simulink model "ExRobotAndEnvironmentControllerContPI"  (Simulink 8.9)
settings: Solver=ode45  StartTime=0.0  StopTime=1000  FixedStep=.01  RelTol=1e-3  EnableMultiTasking=on
undefined symbols (not defined in the file): Env, INITIAL_ROBOT_POS_THETA, INITIAL_ROBOT_POS_X, INITIAL_ROBOT_POS_Y, INTER_WHEEL_DISTANCE, ki_teta, kp_teta, MAX_SPEED, Robot, RobotInit, T, threshold_blanc, threshold_distance, threshold_noir, ts, ts_anim
libraries: simulink x3
settings Model: SuppressorTable=22 serialization::archive 11 0 6 0 0 0 11 0  Creator=alex  LastModifiedBy=esperonb  NumberOfSteps=100
settings OptimizationCC: ExpressionDepthLimit=2147483647
settings SFSimCC: SimParseCustomCode=off

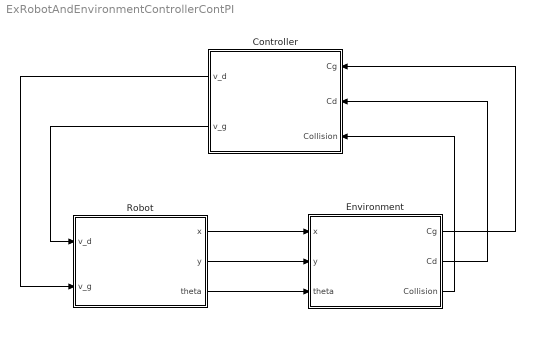
== system ExRobotAndEnvironmentControllerContPI ==
  Controller : Subsystem
  Environment : Subsystem
  Robot : Subsystem
  wires:
  Robot/1(x) -> Environment/1(x)
  Robot/2(y) -> Environment/2(y)
  Robot/3(theta) -> Environment/3(theta)
  Environment/1(Cg) -> Controller/1(Cg)
  Environment/2(Cd) -> Controller/2(Cd)
  Controller/1(v_d) -> Robot/2(v_g)
  Controller/2(v_g) -> Robot/1(v_d)
  Environment/3("Collision ") -> Controller/3("Collision ")

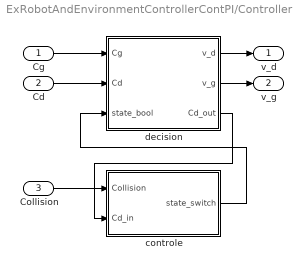
== system ExRobotAndEnvironmentControllerContPI/Controller ==
  Cg : Inport  OutDataTypeStr=double
  Cd : Inport  Port=2  OutDataTypeStr=double
  "Collision " : Inport  Port=3
  controle : Subsystem
  decision : Subsystem
  v_d : Outport
  v_g : Outport  Port=2
  wires:
  "Collision "/1 -> controle/1("Collision ")
  decision/3(Cd_out) -> controle/2(Cd_in)
  controle/1("state_switch ") -> decision/3("state_bool ")
  Cg/1 -> decision/1(Cg)
  Cd/1 -> decision/2(Cd)
  decision/1(v_d) -> v_d/1
  decision/2(v_g) -> v_g/1

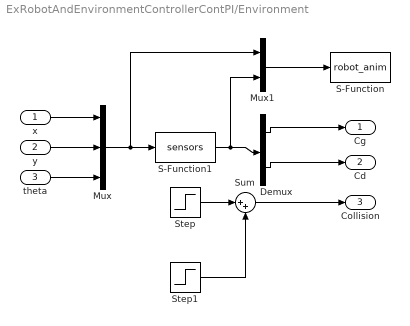
== system ExRobotAndEnvironmentControllerContPI/Environment ==
  x : Inport
  y : Inport  Port=2
  theta : Inport  Port=3
  Demux : Demux  Outputs=2
  Mux : Mux  Inputs=3
  Mux1 : Mux  Inputs=2
  S-Function : S-Function  FunctionName=robot_anim  Parameters=ts_anim,Env,Robot,RobotInit  SFunctionDeploymentMode=off  EnableBusSupport=off
  S-Function1 : S-Function  FunctionName=sensors  Parameters=ts,Env,Robot  SFunctionDeploymentMode=off  EnableBusSupport=off
  Step : Step  Time=2  SampleTime=0
  Step1 : Step  Time=2.1  After=-1  SampleTime=0
  Sum : Sum  Inputs=|++
  Cg : Outport  OutDataTypeStr=double
  Cd : Outport  Port=2
  "Collision " : Outport  Port=3
  wires:
  x/1 -> Mux/1
  y/1 -> Mux/2
  theta/1 -> Mux/3
  Mux/1 -> S-Function1/1, Mux1/1
  S-Function1/1 -> Mux1/2, Demux/1
  Mux1/1 -> S-Function/1
  Demux/1 -> Cg/1
  Demux/2 -> Cd/1
  Sum/1 -> "Collision "/1
  Step/1 -> Sum/1
  Step1/1 -> Sum/2

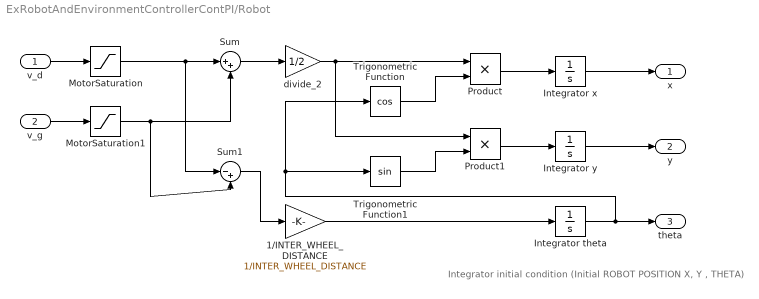
== system ExRobotAndEnvironmentControllerContPI/Robot ==
  note: Integrator initial condition (Initial ROBOT POSITION X, Y , THETA)
  v_d : Inport
  v_g : Inport  Port=2
  1/INTER_WHEEL_DISTANCE : Gain  Gain=1/INTER_WHEEL_DISTANCE
  Integrator theta : Integrator  InitialCondition=INITIAL_ROBOT_POS_THETA
  Integrator x : Integrator  InitialCondition=INITIAL_ROBOT_POS_X
  Integrator y : Integrator  InitialCondition=INITIAL_ROBOT_POS_Y
  MotorSaturation : Saturate  UpperLimit=MAX_SPEED  LowerLimit=-MAX_SPEED
  MotorSaturation1 : Saturate  UpperLimit=MAX_SPEED  LowerLimit=-MAX_SPEED
  Product : Product  RndMeth=Zero
  Product1 : Product  RndMeth=Zero
  Sum : Sum  Inputs=|++
  Sum1 : Sum  Inputs=|-+
  Trigonometric Function : Trigonometry  Operator=cos
  Trigonometric Function1 : Trigonometry
  divide_2 : Gain  Gain=1/2
  x : Outport
  y : Outport  Port=2
  theta : Outport  Port=3
  wires:
  v_d/1 -> MotorSaturation/1
  Integrator x/1 -> x/1
  Integrator y/1 -> y/1
  Integrator theta/1 -> Trigonometric Function/1, Trigonometric Function1/1, theta/1
  Sum/1 -> divide_2/1
  divide_2/1 -> Product1/1, Product/1
  Trigonometric Function/1 -> Product/2
  Trigonometric Function1/1 -> Product1/2
  Product/1 -> Integrator x/1
  Product1/1 -> Integrator y/1
  Sum1/1 -> 1/INTER_WHEEL_DISTANCE/1
  1/INTER_WHEEL_DISTANCE/1 -> Integrator theta/1
  v_g/1 -> MotorSaturation1/1
  MotorSaturation1/1 -> Sum/2, Sum1/2
  MotorSaturation/1 -> Sum/1, Sum1/1

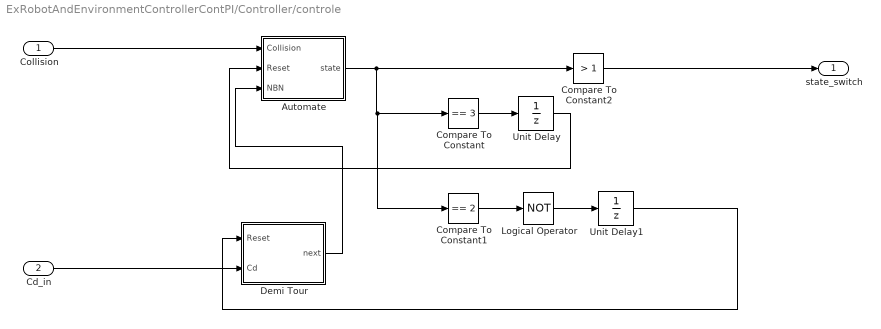
== system ExRobotAndEnvironmentControllerContPI/Controller/controle ==
  "Collision " : Inport
  Cd_in : Inport  Port=2
  Automate : Subsystem
  Compare To Constant : simulink/Logic and Bit Operations/Compare To Constant  relop===  const=3  OutDataTypeStr=boolean
  Compare To Constant1 : simulink/Logic and Bit Operations/Compare To Constant  relop===  const=2  OutDataTypeStr=boolean
  Compare To Constant2 : simulink/Logic and Bit Operations/Compare To Constant  relop=>  const=1  OutDataTypeStr=boolean
  Demi Tour : Subsystem
  Logical Operator : Logic  Operator=NOT  AllPortsSameDT=off  OutDataTypeStr=boolean
  Unit Delay : UnitDelay  SampleTime=-1
  Unit Delay1 : UnitDelay  SampleTime=-1
  "state_switch " : Outport
  wires:
  Cd_in/1 -> Demi Tour/2(Cd)
  "Collision "/1 -> Automate/1(Collision)
  Demi Tour/1(next) -> Automate/3(NBN)
  Automate/1("state ") -> Compare To Constant2/1, Compare To Constant1/1, Compare To Constant/1
  Compare To Constant/1 -> Unit Delay/1
  Compare To Constant1/1 -> Logical Operator/1
  Unit Delay/1 -> Automate/2(Reset)
  Logical Operator/1 -> Unit Delay1/1
  Unit Delay1/1 -> Demi Tour/1(Reset)
  Compare To Constant2/1 -> "state_switch "/1

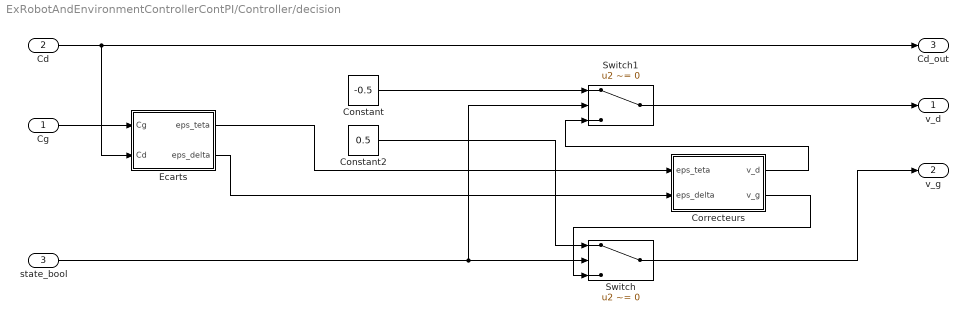
== system ExRobotAndEnvironmentControllerContPI/Controller/decision ==
  Cg : Inport  OutDataTypeStr=double
  Cd : Inport  Port=2  OutDataTypeStr=double
  "state_bool " : Inport  Port=3  OutDataTypeStr=double
  Constant : Constant  Value=-0.5  OutDataTypeStr=double
  Constant2 : Constant  Value=0.5  OutDataTypeStr=double
  "Correcteurs " : Subsystem
  Ecarts : Subsystem
  Switch : Switch  Criteria=u2 ~= 0  Threshold=1
  Switch1 : Switch  Criteria=u2 ~= 0  Threshold=1
  v_d : Outport
  v_g : Outport  Port=2
  Cd_out : Outport  Port=3
  wires:
  "state_bool "/1 -> Switch1/2, Switch/2
  Switch1/1 -> v_d/1
  "Correcteurs "/2(v_g) -> Switch/3
  "Correcteurs "/1(v_d) -> Switch1/3
  Cg/1 -> Ecarts/1(Cg)
  Cd/1 -> Cd_out/1, Ecarts/2(Cd)
  Ecarts/1(eps_teta) -> "Correcteurs "/1(eps_teta)
  Constant/1 -> Switch1/1
  Ecarts/2(eps_delta) -> "Correcteurs "/2(eps_delta)
  Constant2/1 -> Switch/1
  Switch/1 -> v_g/1

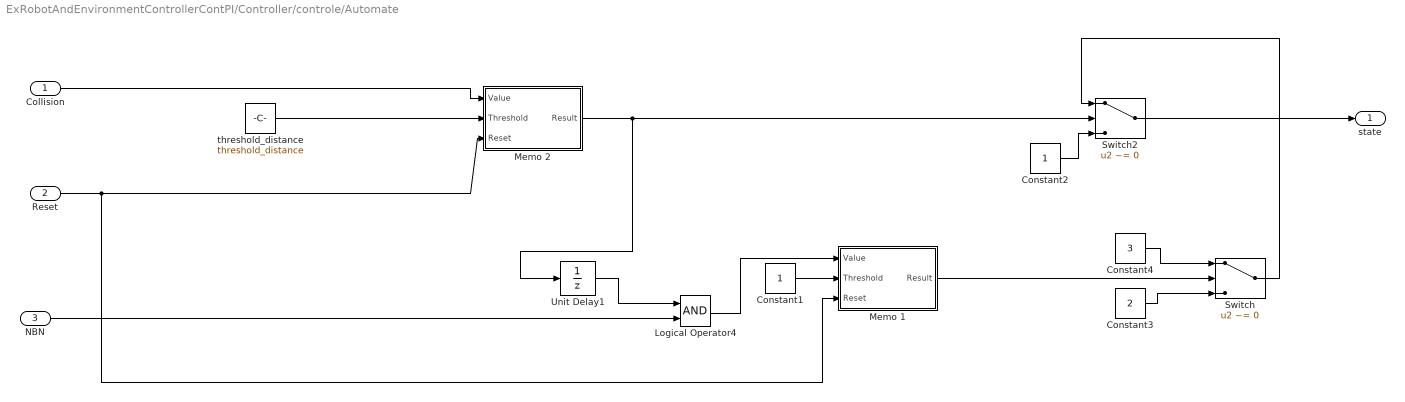
== system ExRobotAndEnvironmentControllerContPI/Controller/controle/Automate ==
  Collision : Inport
  Reset : Inport  Port=2
  NBN : Inport  Port=3
  Constant1 : Constant
  Constant2 : Constant  OutDataTypeStr=uint8
  Constant3 : Constant  Value=2  OutDataTypeStr=uint8
  Constant4 : Constant  Value=3  OutDataTypeStr=uint8
  Logical Operator4 : Logic  AllPortsSameDT=off  OutDataTypeStr=boolean
  Memo 1 : Subsystem
  Memo 2 : Subsystem
  Switch : Switch  Criteria=u2 ~= 0
  Switch2 : Switch  Criteria=u2 ~= 0
  Unit Delay1 : UnitDelay  SampleTime=-1
  threshold_distance : Constant  Value=threshold_distance  OutDataTypeStr=double
  "state " : Outport
  wires:
  Collision/1 -> Memo 2/1(Value)
  Reset/1 -> Memo 1/3(Reset), Memo 2/3(Reset)
  threshold_distance/1 -> Memo 2/2(Threshold)
  Unit Delay1/1 -> Logical Operator4/1
  Logical Operator4/1 -> Memo 1/1(Value)
  NBN/1 -> Logical Operator4/2
  Constant1/1 -> Memo 1/2(Threshold)
  Constant2/1 -> Switch2/3
  Switch2/1 -> "state "/1
  Constant4/1 -> Switch/1
  Constant3/1 -> Switch/3
  Memo 2/1(Result) -> Unit Delay1/1, Switch2/2
  Switch/1 -> Switch2/1
  Memo 1/1(Result) -> Switch/2

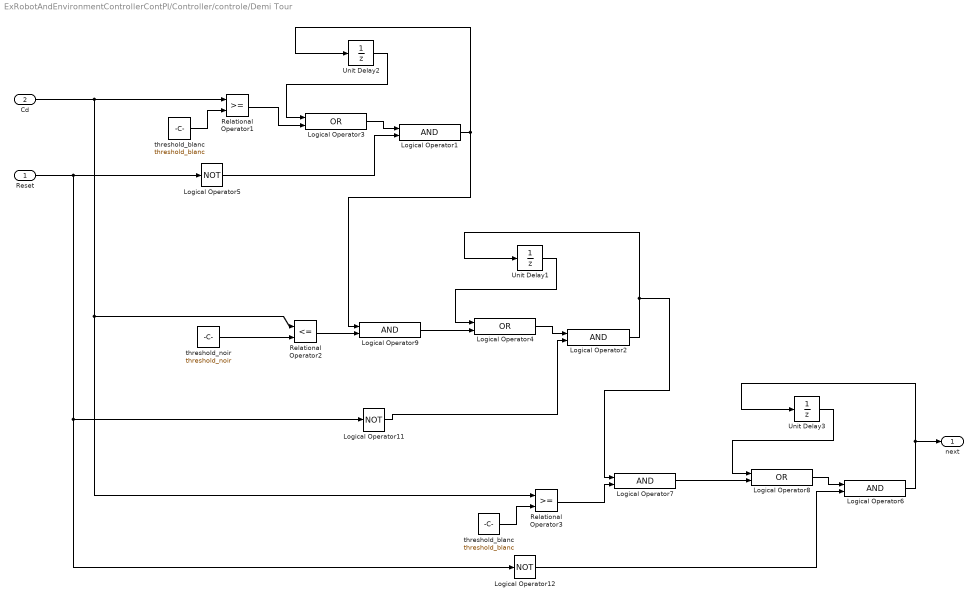
== system ExRobotAndEnvironmentControllerContPI/Controller/controle/Demi Tour ==
  Reset : Inport
  Cd : Inport  Port=2  OutDataTypeStr=double
  Logical Operator{1..2,6..7,9} (5 alike) : Logic  AllPortsSameDT=off  OutDataTypeStr=boolean
  Logical Operator11 : Logic  Operator=NOT  AllPortsSameDT=off  OutDataTypeStr=boolean
  Logical Operator12 : Logic  Operator=NOT  AllPortsSameDT=off  OutDataTypeStr=boolean
  Logical Operator3 : Logic  Operator=OR  AllPortsSameDT=off  OutDataTypeStr=boolean
  Logical Operator4 : Logic  Operator=OR  AllPortsSameDT=off  OutDataTypeStr=boolean
  Logical Operator5 : Logic  Operator=NOT  AllPortsSameDT=off  OutDataTypeStr=boolean
  Logical Operator8 : Logic  Operator=OR  AllPortsSameDT=off  OutDataTypeStr=boolean
  Relational Operator1 : RelationalOperator  OutDataTypeStr=boolean  RndMeth=Simplest
  Relational Operator2 : RelationalOperator  Operator=<=  OutDataTypeStr=boolean  RndMeth=Simplest
  Relational Operator3 : RelationalOperator  OutDataTypeStr=boolean  RndMeth=Simplest
  Unit Delay1 : UnitDelay  SampleTime=-1
  Unit Delay2 : UnitDelay  SampleTime=-1
  Unit Delay3 : UnitDelay  SampleTime=-1
  threshold_blanc : Constant  Value=threshold_blanc  OutDataTypeStr=double
  "threshold_blanc " : Constant  Value=threshold_blanc  OutDataTypeStr=double
  threshold_noir : Constant  Value=threshold_noir  OutDataTypeStr=double
  next : Outport
  wires:
  Logical Operator5/1 -> Logical Operator1/2
  Reset/1 -> Logical Operator5/1, Logical Operator11/1, Logical Operator12/1
  "threshold_blanc "/1 -> Relational Operator1/2
  Relational Operator2/1 -> Logical Operator9/2
  threshold_noir/1 -> Relational Operator2/2
  Cd/1 -> Relational Operator3/1, Relational Operator2/1, Relational Operator1/1
  Relational Operator3/1 -> Logical Operator7/2
  threshold_blanc/1 -> Relational Operator3/2
  Logical Operator3/1 -> Logical Operator1/1
  Relational Operator1/1 -> Logical Operator3/2
  Logical Operator1/1 -> Unit Delay2/1, Logical Operator9/1
  Unit Delay2/1 -> Logical Operator3/1
  Logical Operator2/1 -> Logical Operator7/1, Unit Delay1/1
  Unit Delay1/1 -> Logical Operator4/1
  Logical Operator4/1 -> Logical Operator2/1
  Logical Operator9/1 -> Logical Operator4/2
  Logical Operator11/1 -> Logical Operator2/2
  Logical Operator8/1 -> Logical Operator6/1
  Logical Operator7/1 -> Logical Operator8/2
  Unit Delay3/1 -> Logical Operator8/1
  Logical Operator12/1 -> Logical Operator6/2
  Logical Operator6/1 -> next/1, Unit Delay3/1

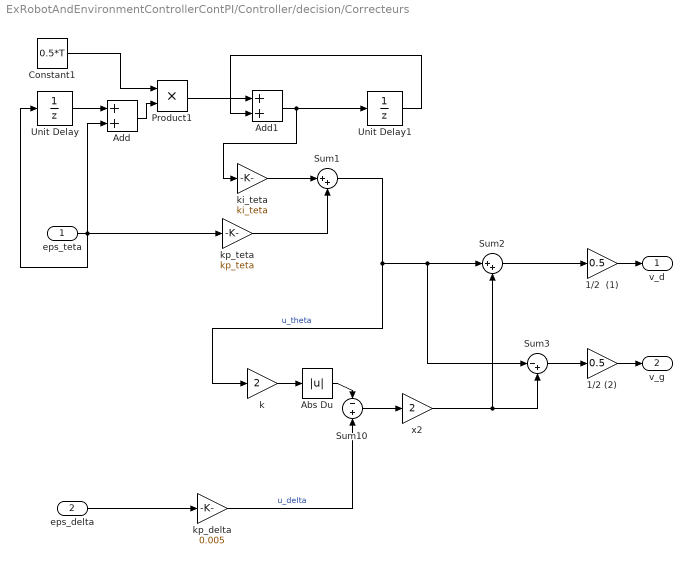
== system ExRobotAndEnvironmentControllerContPI/Controller/decision/Correcteurs  ==
  eps_teta : Inport
  eps_delta : Inport  Port=2
  1/2  (1) : Gain  Gain=0.5  SaturateOnIntegerOverflow=on  OutDataTypeStr=Inherit: Same as input  ParamDataTypeStr=Inherit: Same as input
  1/2 (2) : Gain  Gain=0.5  SaturateOnIntegerOverflow=on  OutDataTypeStr=Inherit: Same as input  ParamDataTypeStr=Inherit: Same as input
  Abs Du : Abs  SaturateOnIntegerOverflow=on
  Add : Sum
  Add1 : Sum
  Constant1 : Constant  Value=0.5*T
  Product1 : Product
  Sum1 : Sum  Inputs=|++  SaturateOnIntegerOverflow=on
  Sum10 : Sum  Inputs=-+  SaturateOnIntegerOverflow=on
  Sum2 : Sum  Inputs=|++  SaturateOnIntegerOverflow=on
  Sum3 : Sum  Inputs=|-+  SaturateOnIntegerOverflow=on
  Unit Delay : UnitDelay  SampleTime=-1
  Unit Delay1 : UnitDelay  SampleTime=-1
  k : Gain  Gain=2  SaturateOnIntegerOverflow=on  OutDataTypeStr=Inherit: Same as input  ParamDataTypeStr=Inherit: Same as input
  ki_teta : Gain  Gain=ki_teta  SaturateOnIntegerOverflow=on  OutDataTypeStr=Inherit: Same as input  ParamDataTypeStr=Inherit: Same as input
  kp_delta : Gain  Gain=0.005
  kp_teta : Gain  Gain=kp_teta  SaturateOnIntegerOverflow=on  OutDataTypeStr=Inherit: Same as input  ParamDataTypeStr=Inherit: Same as input
  x2 : Gain  Gain=2  SaturateOnIntegerOverflow=on  OutDataTypeStr=Inherit: Same as input  ParamDataTypeStr=Inherit: Same as input
  v_d : Outport
  v_g : Outport  Port=2
  wires:
  ki_teta/1 -> Sum1/1
  kp_teta/1 -> Sum1/2
  Sum2/1 -> 1/2  (1)/1
  Sum3/1 -> 1/2 (2)/1
  k/1 -> Abs Du/1
  kp_delta/1 -> Sum10/2  "u_delta"
  eps_teta/1 -> Add/2, Unit Delay/1, kp_teta/1
  Abs Du/1 -> Sum10/1
  x2/1 -> Sum2/2, Sum3/2
  Sum10/1 -> x2/1
  Sum1/1 -> k/1, Sum2/1, Sum3/1  "u_theta"
  1/2  (1)/1 -> v_d/1
  1/2 (2)/1 -> v_g/1
  eps_delta/1 -> kp_delta/1
  Add1/1 -> Unit Delay1/1, ki_teta/1
  Unit Delay/1 -> Add/1
  Add/1 -> Product1/2
  Constant1/1 -> Product1/1
  Product1/1 -> Add1/1
  Unit Delay1/1 -> Add1/2

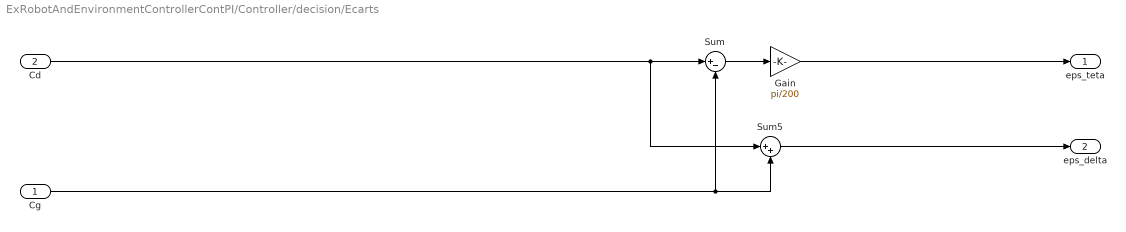
== system ExRobotAndEnvironmentControllerContPI/Controller/decision/Ecarts ==
  Cg : Inport  OutDataTypeStr=double
  Cd : Inport  Port=2  OutDataTypeStr=double
  Gain : Gain  Gain=pi/200
  Sum : Sum  Inputs=|+-
  Sum5 : Sum  Inputs=|++
  eps_teta : Outport
  eps_delta : Outport  Port=2
  wires:
  Sum/1 -> Gain/1
  Cd/1 -> Sum/1, Sum5/1
  Cg/1 -> Sum/2, Sum5/2
  Gain/1 -> eps_teta/1
  Sum5/1 -> eps_delta/1

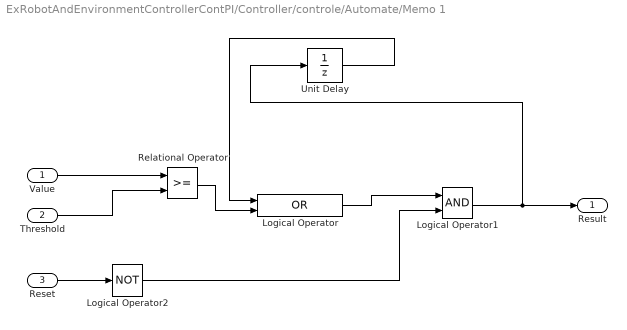
== system ExRobotAndEnvironmentControllerContPI/Controller/controle/Automate/Memo 1 ==
  Value : Inport
  Threshold : Inport  Port=2
  Reset : Inport  Port=3
  Logical Operator : Logic  Operator=OR  AllPortsSameDT=off  OutDataTypeStr=boolean
  Logical Operator1 : Logic  AllPortsSameDT=off  OutDataTypeStr=boolean
  Logical Operator2 : Logic  Operator=NOT  AllPortsSameDT=off  OutDataTypeStr=boolean
  Relational Operator : RelationalOperator  OutDataTypeStr=boolean  RndMeth=Simplest
  Unit Delay : UnitDelay  SampleTime=-1
  Result : Outport
  wires:
  Reset/1 -> Logical Operator2/1
  Relational Operator/1 -> Logical Operator/2
  Threshold/1 -> Relational Operator/2
  Logical Operator2/1 -> Logical Operator1/2
  Logical Operator1/1 -> Unit Delay/1, Result/1
  Value/1 -> Relational Operator/1
  Logical Operator/1 -> Logical Operator1/1
  Unit Delay/1 -> Logical Operator/1

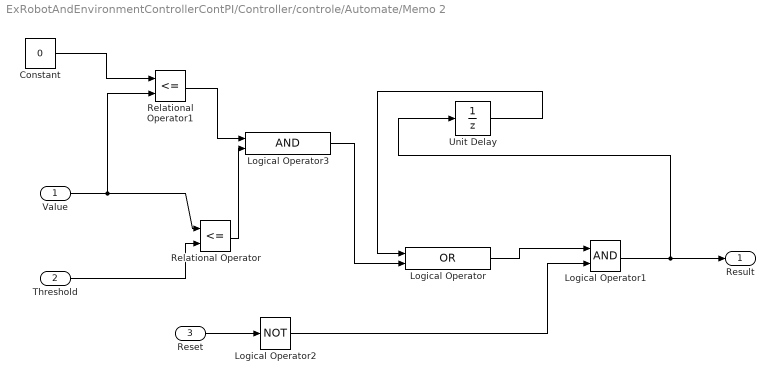
== system ExRobotAndEnvironmentControllerContPI/Controller/controle/Automate/Memo 2 ==
  Value : Inport
  Threshold : Inport  Port=2
  Reset : Inport  Port=3
  Constant : Constant  Value=0
  Logical Operator : Logic  Operator=OR  AllPortsSameDT=off  OutDataTypeStr=boolean
  Logical Operator1 : Logic  AllPortsSameDT=off  OutDataTypeStr=boolean
  Logical Operator2 : Logic  Operator=NOT  AllPortsSameDT=off  OutDataTypeStr=boolean
  Logical Operator3 : Logic  AllPortsSameDT=off  OutDataTypeStr=boolean
  Relational Operator : RelationalOperator  Operator=<=  OutDataTypeStr=boolean  RndMeth=Simplest
  Relational Operator1 : RelationalOperator  Operator=<=  OutDataTypeStr=boolean  RndMeth=Simplest
  Unit Delay : UnitDelay  SampleTime=-1
  Result : Outport
  wires:
  Reset/1 -> Logical Operator2/1
  Threshold/1 -> Relational Operator/2
  Logical Operator2/1 -> Logical Operator1/2
  Logical Operator1/1 -> Unit Delay/1, Result/1
  Value/1 -> Relational Operator1/2, Relational Operator/1
  Logical Operator/1 -> Logical Operator1/1
  Unit Delay/1 -> Logical Operator/1
  Relational Operator/1 -> Logical Operator3/2
  Logical Operator3/1 -> Logical Operator/2
  Relational Operator1/1 -> Logical Operator3/1
  Constant/1 -> Relational Operator1/1
